simulink model "sixDoFDynamics_th"  (R2018b)
settings: Solver=VariableStepAuto  StartTime=0.0  StopTime=10.0  RelTol=1e-3
values from neighbouring files (symbols this model uses):
  FNetBdy = [0;0;-10]    [sixDoFDynamics_ts.m]
  MNetBdy = [0;0;0]    [sixDoFDynamics_ts.m]
libraries: sixDoFDynamics_ul x1
settings Model: Creator=asiddiq2  LastModifiedBy=asiddiq2

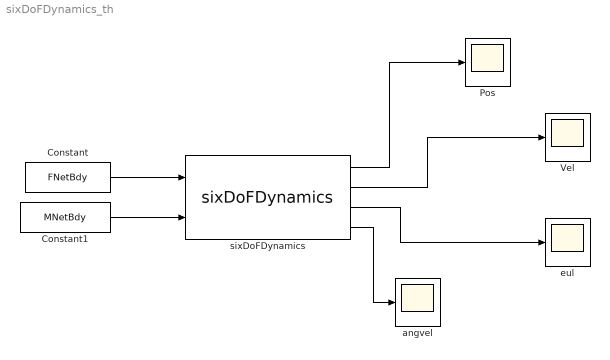
== system sixDoFDynamics_th ==
  Constant : Constant  Value=FNetBdy
  Constant1 : Constant  Value=MNetBdy
  Pos : Scope
  Vel : Scope
  angvel : Scope
  eul : Scope
  sixDoFDynamics : sixDoFDynamics_ul/sixDoFDynamics  massBdy=base_mass  massAdded=added_mass  bdy_MI_cm=MI  initPosCM=ini_pos  initVelCM=ini_vel  initEulAngs=ini_eul  initAngVel=ini_OwB
  wires:
  sixDoFDynamics/1 -> Pos/1
  sixDoFDynamics/4 -> angvel/1
  sixDoFDynamics/3 -> eul/1
  sixDoFDynamics/2 -> Vel/1
  Constant/1 -> sixDoFDynamics/1
  Constant1/1 -> sixDoFDynamics/2
